simulink model "m_control_05"  (R2013b)
settings: Solver=ode45  StartTime=0.0  StopTime=10.0  RelTol=1e-3
settings Model: Creator=Administrator  LastModifiedBy=Administrator

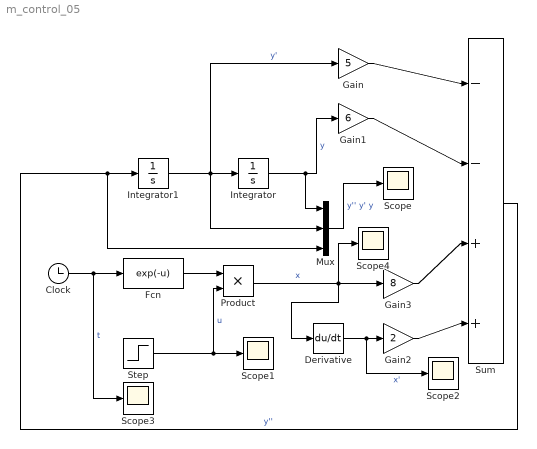
== system m_control_05 ==
  Clock : Clock
  Derivative : Derivative
  Fcn : Fcn  Expr=exp(-u)
      mask Display: disp('exp(-t)');
  Gain : Gain  Gain=5
  Gain1 : Gain  Gain=6
  Gain2 : Gain  Gain=2
  Gain3 : Gain  Gain=8
  Integrator : Integrator  InitialCondition=5
      settings: AttributesFormatString=InitVal = %<InitialCondition>
  Integrator1 : Integrator  InitialCondition=-4
      settings: AttributesFormatString=InitVal = %<InitialCondition>
  Mux : Mux  Inputs=3
  Product : Product
  Scope{,1..4} (5 alike) : Scope
      Scope2 settings: SaveName=ScopeData2
      Scope3 settings: SaveName=ScopeData3
      Scope4 settings: SaveName=ScopeData4
  Step : Step  Time=4  SampleTime=0
  Sum : Sum  Inputs=--||++
  wires:
  Integrator1/1 -> Mux/2, Gain/1, Integrator/1  "y'"
  Sum/1 -> Mux/3, Integrator1/1  "y''"
  Integrator/1 -> Mux/1, Gain1/1  "y"
  Clock/1 -> Scope3/1, Fcn/1  "t"
  Fcn/1 -> Product/1
  Step/1 -> Scope1/1, Product/2  "u"
  Product/1 -> Derivative/1, Scope4/1, Gain3/1  "x"
  Derivative/1 -> Scope2/1, Gain2/1  "x'"
  Gain2/1 -> Sum/4
  Gain3/1 -> Sum/3
  Gain/1 -> Sum/1
  Gain1/1 -> Sum/2
  Mux/1 -> Scope/1  "y'' y' y"
